simulink model "qdr_ct_test4"  (R2013b)
settings: Solver=FixedStepDiscrete  SolverMode=SingleTasking  StartTime=0.0  StopTime=1000.0  RelTol=1e-3
libraries: xbsIndex_r4 x636, casper_library_delays x8, xps_library x7, casper_library_misc x7
(part 1 of 8)
settings Model: Creator=franco  LastModifiedBy=root

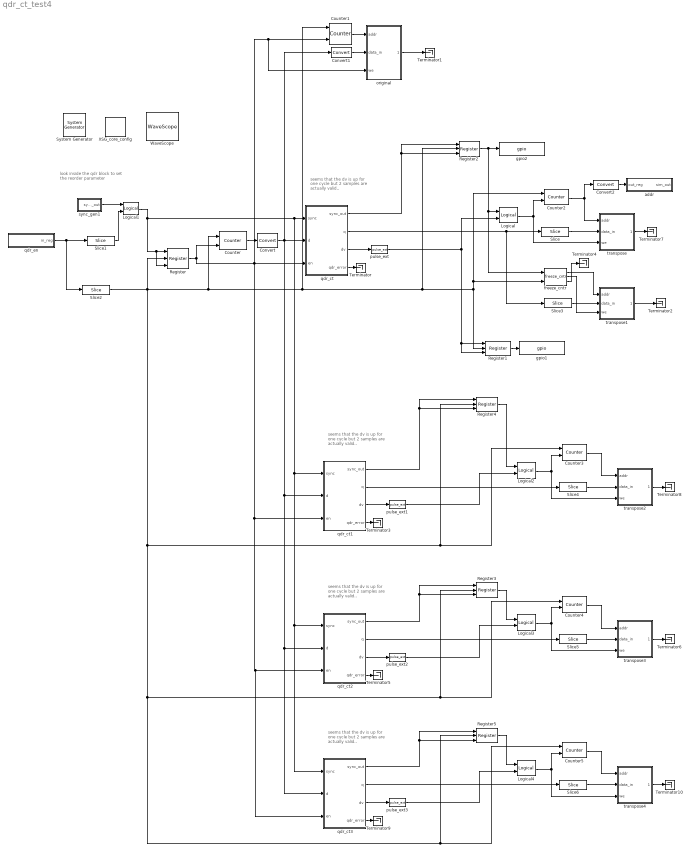
== system qdr_ct_test4 ==
  note: seems that the dv
      | is up for one cycle
      | but 2 samples are
      | actually valid..
  note: look inside the qdr block
      | to set the reorder parameter
  note: seems that the dv
      | is up for one cycle
      | but 2 samples are
      | actually valid..
  note: seems that the dv
      | is up for one cycle
      | but 2 samples are
      | actually valid..
  note: seems that the dv
      | is up for one cycle
      | but 2 samples are
      | actually valid..
  " System Generator" : xbsIndex_r4/ System Generator  Tag=genX  xilinxfamily=virtex6  part=xc6vsx475t  speed=-1  package=ff1759  synthesis_tool=XST  clock_wrapper=Clock Enables  directory=./qdr_ct_test/sysgen  proj_type=Project Navigator  Synth_file=XST Defaults  Impl_file=ISE Defaults  testbench=off  simulink_period=1  sysclk_period=7.4074  dcm_input_clock_period=100  incr_netlist=off  trim_vbits=Everywhere in SubSystem  dbl_ovrd=According to Block Masks  core_generation=According to Block Masks  run_coregen=off  deprecated_control=off  eval_field=0  block_type=sysgen
  Convert : xbsIndex_r4/Convert  gui_display_data_type=Fixed-point  arith_type=Unsigned  n_bits=72  bin_pt=0  float_type=Single  exp_bits=8  fraction_bits=24  quantization=Truncate  overflow=Wrap  en=off  latency=0  dbl_ovrd=off  pipeline=off  block_type=convert
  Convert1 : xbsIndex_r4/Convert  gui_display_data_type=Fixed-point  arith_type=Unsigned  n_bits=32  bin_pt=0  float_type=Single  exp_bits=8  fraction_bits=24  quantization=Truncate  overflow=Wrap  en=off  latency=0  dbl_ovrd=off  pipeline=off  block_type=convert
  Convert2 : xbsIndex_r4/Convert  gui_display_data_type=Fixed-point  arith_type=Unsigned  n_bits=32  bin_pt=0  float_type=Single  exp_bits=8  fraction_bits=24  quantization=Truncate  overflow=Wrap  en=off  latency=2  dbl_ovrd=off  pipeline=off  block_type=convert
      settings: block_version=11.4
  Counter{,1..5} (6 alike) : xbsIndex_r4/Counter  cnt_type=Free Running  cnt_to=Inf  operation=Up  start_count=0  cnt_by_val=1  arith_type=Unsigned  n_bits=16  bin_pt=0  load_pin=off  rst=on  en=on  explicit_period=on  period=1  dbl_ovrd=off  use_behavioral_HDL=off  implementation=Fabric  block_type=counter
  Logical{,1..4} (5 alike) : xbsIndex_r4/Logical  logical_function=AND  inputs=2  en=off  latency=0  precision=Full  arith_type=Unsigned  n_bits=16  bin_pt=0  align_bp=on  dbl_ovrd=off  block_type=logical
  Register{,1..5} (6 alike) : xbsIndex_r4/Register  init=0  rst=on  en=on  dbl_ovrd=off  block_type=register
  Slice{,3..6} (5 alike) : xbsIndex_r4/Slice  nbits=32  boolean_output=off  mode=Lower Bit Location + Width  bit1=0  base1=MSB of Input  bit0=0  base0=LSB of Input  dbl_ovrd=off  block_type=slice
  Slice1 : xbsIndex_r4/Slice  nbits=1  boolean_output=on  mode=Lower Bit Location + Width  bit1=0  base1=MSB of Input  bit0=0  base0=LSB of Input  dbl_ovrd=off  block_type=slice
  Slice2 : xbsIndex_r4/Slice  nbits=1  boolean_output=on  mode=Lower Bit Location + Width  bit1=0  base1=MSB of Input  bit0=1  base0=LSB of Input  dbl_ovrd=off  block_type=slice
  Terminator{,1..10} (11 alike) : Terminator
  WaveScope : xbsIndex_r4/WaveScope  block_type=wavescope
  XSG_core_config : xps_library/XSG_core_config  Tag=xps:xsg  hw_sys=ROACH2:sx475t  clk_src=sys_clk  ROACH_clk_src=sys_clk  ROACH2_clk_src=sys_clk  MKDIG_clk_src=sys_clk  clk_rate=135  sample_period=1  synthesis_tool=XST
  addr : Subsystem  Tag=xps:sw_reg  AncestorBlock=xps_library/software_register  mask(swreg){io_dir=To Processor, io_delay=0, sample_period=1, names=reg, bitwidths=32, bin_pts=0, arith_types=0, sim_port=on, show_format=on}
      mask prompts: io_dir "I/O direction"; io_delay "I/O delay"; sample_period "Sample period"; names "Bitfield names [msb...lsb]"; bitwidths "Bitfield widths"; bin_pts "Bitfield binary pts"; arith_types "Bitfield types, ufix=0, fix=1, bool=2"; sim_port "Provide sim input/output?"; show_format "Print format string?"
      mask help: A 32-bit software-accessible register. Can be divided into bitfields of varying widths and types using the fields in the block mask.
      mask init:
      | try
      |     swreg_init(gcb)
      | catch ex
      |     disp(sprintf('%s: %s', gcb, ex.message))
      |     errordlg(ex.message)
      | end
      settings: AttributesFormatString=1output:uf32.0 = 32 bits
      mask TypeOptions io_dir: To Processor | From Processor
      mask Callback io_dir:
      | mask_enables = get_param(gcb, 'MaskEnables');
      | mask_names = get_param(gcb, 'MaskNames');
      | if strcmp(get_param(gcb, 'io_dir'), 'To Processor'),
      |     mask_enables{ismember(mask_names, 'sample_period')} = 'off';
      | else
      |     mask_enables{ismember(mask_names, 'sample_period')} = 'on';
      | end
      | set_param(gcb, 'MaskEnables', mask_enables);
  freeze_cntr : casper_library_misc/freeze_cntr  CounterBits=16
  gpio1 : xps_library/gpio  Tag=xps:gpio  io_group=ROACH2:led  io_dir=out  arith_type=Boolean  bitwidth=1  bin_pt=0  bit_index=1  sample_period=1  use_single_ended=off  use_ddr=off  reg_iob=on  reg_clk_phase=0  termination=None
  gpio2 : xps_library/gpio  Tag=xps:gpio  io_group=ROACH2:led  io_dir=out  arith_type=Boolean  bitwidth=1  bin_pt=0  bit_index=0  sample_period=1  use_single_ended=off  use_ddr=off  reg_iob=on  reg_clk_phase=0  termination=None
  original : Subsystem  Tag=xps:bram  AncestorBlock=xps_library/Shared_BRAM  mask{arith_type=Unsigned, addr_width=16, data_width=32, reg_prim_output=off, reg_core_output=off, optimization=Minimum_Area, data_bin_pt=0, init_vals=[0:2^10-1], sample_rate=1}
      mask prompts: arith_type "Output Data Type"; addr_width "Address width"; data_width "Data Width"; reg_prim_output "Register Primitive Output"; reg_core_output "Register Core Output"; data_bin_pt "Data Binary Point"; init_vals "Initial values (simulation only)"; sample_rate "Sample rate"
      mask init:
      | shared_bram_mask;
      mask TypeOptions arith_type: Unsigned | Signed  (2's comp)
      mask TypeOptions data_width: 8 | 16 | 32 | 64 | 128
      mask TypeOptions optimization: Minimum_Area | Low_Power
  pulse_ext{,1..3} (4 alike) : casper_library_misc/pulse_ext  pulse_len=2
  qdr_ct : Subsystem  AncestorBlock=casper_library_reorder/qdr_ct  mask{idepth=8, odepth=8, which_qdr=qdr0, swap_input=no, output_order=in order, step_bits=0, custom_map=[1  15   5   7  10  14   6   0   8   9   2  13  12  11   4   3]}
      mask prompts: idepth "Input vector length (2^?)"; odepth "Output vector length (2^?)"; which_qdr "QDR SRAM chip"; swap_input "Swap input halves?"; output_order "Output column order"; step_bits "Interleave step (2^?)"; custom_map "Custom map"
      mask help:
      | Writes vectors in as rows in matrix and reads
      | out columns. Order in which columns read out
      | determined by 'Output column order' parameter.
      mask init:
      | if (strcmp(output_order, 'interleaved') == 1) && (step_bits > (idepth-1)) ,
      |     errmsg = sprintf('Can''t make step size (%i) bigger than (input vector bit size (%i) - 1)', step_bits, idepth);
      |     errordlg(errmsg);
      | end    
      | 
      | if strcmp(output_order, 'custom') && (...
      |         length(unique(custom_map)) ~= 2^idepth ||...
      |         ~isempty(find(custom_map < 0)) || ...
      |         ~isempty(find(custom_map > (2^idepth)-1))),
      |     disp('Custom map elements must be unique in range 0->2^(input vector)-1');
      |     return;
      | end
      | 
      | % set up output order (in order, interleaved, or custom)
      | map = 0 : (2^idepth)-1;
      | if strcmp(swap_input, 'yes'),
      |     map = [map((length(map)/2)+1:end), map(1:length(map)/2)];
      | end
      | if strcmp(output_order, 'interleaved'),
      |     index = zeros(1, 2^idepth);
      |     step_size = 2^(idepth-step_bits);
      |     for ctr = 0:(2^step_bits)-1,
      |         start = (ctr * step_size) + 1;
      |         finish = start + step_size - 1;
      |         index(start:finish) = ctr+1 : 2^step_bits : 2^idepth;
      |     end
      |     map = map(index);
      |     clear index;
      | elseif strcmp(output_order, 'custom'),
      |     map = map(custom_map+1);
      | end
      | 
      | %generate map so that two samples from same position in 
      | %subsequent input vectors are written into same address
      | map = reshape([map; 2^idepth+map], 1, 2^(idepth+1));
      | 
      | set_param([gcb, '/reorder'], ...
      |     'map', ['[',num2str(map),']']);
      | set_param([gcb, '/qdr'], 'which_qdr', which_qdr);
      mask TypeOptions which_qdr: qdr0 | qdr1 | qdr2 | qdr3
      mask TypeOptions swap_input: no | yes
      mask TypeOptions output_order: in order | interleaved | custom
  qdr_ct1 : Subsystem  AncestorBlock=casper_library_reorder/qdr_ct  mask{idepth=8, odepth=8, which_qdr=qdr1, swap_input=no, output_order=in order, step_bits=0, custom_map=[1  15   5   7  10  14   6   0   8   9   2  13  12  11   4   3]}
      mask prompts: idepth "Input vector length (2^?)"; odepth "Output vector length (2^?)"; which_qdr "QDR SRAM chip"; swap_input "Swap input halves?"; output_order "Output column order"; step_bits "Interleave step (2^?)"; custom_map "Custom map"
      mask help:
      | Writes vectors in as rows in matrix and reads
      | out columns. Order in which columns read out
      | determined by 'Output column order' parameter.
      mask init: same as qdr_ct_test4/qdr_ct
      mask TypeOptions which_qdr: qdr0 | qdr1 | qdr2 | qdr3
      mask TypeOptions swap_input: no | yes
      mask TypeOptions output_order: in order | interleaved | custom
  qdr_ct2 : Subsystem  AncestorBlock=casper_library_reorder/qdr_ct  mask{idepth=8, odepth=8, which_qdr=qdr2, swap_input=no, output_order=in order, step_bits=0, custom_map=[1  15   5   7  10  14   6   0   8   9   2  13  12  11   4   3]}
      mask prompts: idepth "Input vector length (2^?)"; odepth "Output vector length (2^?)"; which_qdr "QDR SRAM chip"; swap_input "Swap input halves?"; output_order "Output column order"; step_bits "Interleave step (2^?)"; custom_map "Custom map"
      mask help:
      | Writes vectors in as rows in matrix and reads
      | out columns. Order in which columns read out
      | determined by 'Output column order' parameter.
      mask init: same as qdr_ct_test4/qdr_ct
      mask TypeOptions which_qdr: qdr0 | qdr1 | qdr2 | qdr3
      mask TypeOptions swap_input: no | yes
      mask TypeOptions output_order: in order | interleaved | custom
  qdr_ct3 : Subsystem  AncestorBlock=casper_library_reorder/qdr_ct  mask{idepth=8, odepth=8, which_qdr=qdr3, swap_input=no, output_order=in order, step_bits=0, custom_map=[1  15   5   7  10  14   6   0   8   9   2  13  12  11   4   3]}
      mask prompts: idepth "Input vector length (2^?)"; odepth "Output vector length (2^?)"; which_qdr "QDR SRAM chip"; swap_input "Swap input halves?"; output_order "Output column order"; step_bits "Interleave step (2^?)"; custom_map "Custom map"
      mask help:
      | Writes vectors in as rows in matrix and reads
      | out columns. Order in which columns read out
      | determined by 'Output column order' parameter.
      mask init: same as qdr_ct_test4/qdr_ct
      mask TypeOptions which_qdr: qdr0 | qdr1 | qdr2 | qdr3
      mask TypeOptions swap_input: no | yes
      mask TypeOptions output_order: in order | interleaved | custom
  qdr_en : Subsystem  Tag=xps:sw_reg  AncestorBlock=xps_library/software_register  mask(swreg){io_dir=From Processor, io_delay=0, sample_period=1, names=reg, bitwidths=32, bin_pts=0, arith_types=0, sim_port=off, show_format=off}
      mask prompts: io_dir "I/O direction"; io_delay "I/O delay"; sample_period "Sample period"; names "Bitfield names [msb...lsb]"; bitwidths "Bitfield widths"; bin_pts "Bitfield binary pts"; arith_types "Bitfield types, ufix=0, fix=1, bool=2"; sim_port "Provide sim input/output?"; show_format "Print format string?"
      mask help: A 32-bit software-accessible register. Can be divided into bitfields of varying widths and types using the fields in the block mask.
      mask init:
      | try
      |     swreg_init(gcb)
      | catch ex
      |     disp(sprintf('%s: %s', gcb, ex.message))
      |     errordlg(ex.message)
      | end
      settings: AttributesFormatString=1input
      mask TypeOptions io_dir: To Processor | From Processor
      mask Callback io_dir:
      | mask_enables = get_param(gcb, 'MaskEnables');
      | mask_names = get_param(gcb, 'MaskNames');
      | if strcmp(get_param(gcb, 'io_dir'), 'To Processor'),
      |     mask_enables{ismember(mask_names, 'sample_period')} = 'off';
      | else
      |     mask_enables{ismember(mask_names, 'sample_period')} = 'on';
      | end
      | set_param(gcb, 'MaskEnables', mask_enables);
  sync_gen1 : Subsystem  AncestorBlock=casper_library_misc/sync_gen  mask(sync_gen){sim_acc_len=1, fft_size=2^16, fft_simult_inputs=1, pfb_fir_taps=1, reorder_vec=9, scale=1}
      mask prompts: sim_acc_len "Simulation Accumulation Length"; fft_size "FFT Size"; fft_simult_inputs "Simultaneous Inputs (FFT)"; pfb_fir_taps "Taps in pfb_fir (use 1 if no pfb_fir)"; reorder_vec "Reorder Orders (e.g. [2 2 2])"
      mask help:
      | This block computes the sync period based on system parameters as
      | described in Casper memo.  Detailed descritions of the block's
      | variables can be found in the 'Block Documentation' section of
      | the CASPER wiki.
      mask init:
      | sync_gen_init(gcb, ...
      |     'sim_acc_len', sim_acc_len, ...
      |     'fft_size', fft_size, ...
      |     'fft_simult_inputs', fft_simult_inputs,...
      |     'pfb_fir_taps', pfb_fir_taps, ...
      |     'reorder_vec', reorder_vec, ...
      |     'scale', scale);
      settings: AttributesFormatString=sim_sync_period=589824
      mask Help:
      | SyncPeriod=LCM(reorder_vec)*(acc_num)*(pfb_fir_len)*(fft_size/fft_simult_inputs)
      | 
      | See CASPER sync pulse memo for more details.
  transpose : Subsystem  Tag=xps:bram  AncestorBlock=xps_library/Shared_BRAM  mask{arith_type=Unsigned, addr_width=16, data_width=32, reg_prim_output=off, reg_core_output=off, optimization=Minimum_Area, data_bin_pt=0, init_vals=[0:2^10-1], sample_rate=1}
      mask prompts: arith_type "Output Data Type"; addr_width "Address width"; data_width "Data Width"; reg_prim_output "Register Primitive Output"; reg_core_output "Register Core Output"; data_bin_pt "Data Binary Point"; init_vals "Initial values (simulation only)"; sample_rate "Sample rate"
      mask init:
      | shared_bram_mask;
      mask TypeOptions arith_type: Unsigned | Signed  (2's comp)
      mask TypeOptions data_width: 8 | 16 | 32 | 64 | 128
      mask TypeOptions optimization: Minimum_Area | Low_Power
  transpose1 : Subsystem  Tag=xps:bram  AncestorBlock=xps_library/Shared_BRAM  mask{arith_type=Unsigned, addr_width=16, data_width=32, reg_prim_output=off, reg_core_output=off, optimization=Minimum_Area, data_bin_pt=0, init_vals=[0:2^10-1], sample_rate=1}
      mask prompts: arith_type "Output Data Type"; addr_width "Address width"; data_width "Data Width"; reg_prim_output "Register Primitive Output"; reg_core_output "Register Core Output"; data_bin_pt "Data Binary Point"; init_vals "Initial values (simulation only)"; sample_rate "Sample rate"
      mask init:
      | shared_bram_mask;
      mask TypeOptions arith_type: Unsigned | Signed  (2's comp)
      mask TypeOptions data_width: 8 | 16 | 32 | 64 | 128
      mask TypeOptions optimization: Minimum_Area | Low_Power
  transpose2 : Subsystem  Tag=xps:bram  AncestorBlock=xps_library/Shared_BRAM  mask{arith_type=Unsigned, addr_width=16, data_width=32, reg_prim_output=off, reg_core_output=off, optimization=Minimum_Area, data_bin_pt=0, init_vals=[0:2^10-1], sample_rate=1}
      mask prompts: arith_type "Output Data Type"; addr_width "Address width"; data_width "Data Width"; reg_prim_output "Register Primitive Output"; reg_core_output "Register Core Output"; data_bin_pt "Data Binary Point"; init_vals "Initial values (simulation only)"; sample_rate "Sample rate"
      mask init:
      | shared_bram_mask;
      mask TypeOptions arith_type: Unsigned | Signed  (2's comp)
      mask TypeOptions data_width: 8 | 16 | 32 | 64 | 128
      mask TypeOptions optimization: Minimum_Area | Low_Power
  transpose3 : Subsystem  Tag=xps:bram  AncestorBlock=xps_library/Shared_BRAM  mask{arith_type=Unsigned, addr_width=16, data_width=32, reg_prim_output=off, reg_core_output=off, optimization=Minimum_Area, data_bin_pt=0, init_vals=[0:2^10-1], sample_rate=1}
      mask prompts: arith_type "Output Data Type"; addr_width "Address width"; data_width "Data Width"; reg_prim_output "Register Primitive Output"; reg_core_output "Register Core Output"; data_bin_pt "Data Binary Point"; init_vals "Initial values (simulation only)"; sample_rate "Sample rate"
      mask init:
      | shared_bram_mask;
      mask TypeOptions arith_type: Unsigned | Signed  (2's comp)
      mask TypeOptions data_width: 8 | 16 | 32 | 64 | 128
      mask TypeOptions optimization: Minimum_Area | Low_Power
  transpose4 : Subsystem  Tag=xps:bram  AncestorBlock=xps_library/Shared_BRAM  mask{arith_type=Unsigned, addr_width=16, data_width=32, reg_prim_output=off, reg_core_output=off, optimization=Minimum_Area, data_bin_pt=0, init_vals=[0:2^10-1], sample_rate=1}
      mask prompts: arith_type "Output Data Type"; addr_width "Address width"; data_width "Data Width"; reg_prim_output "Register Primitive Output"; reg_core_output "Register Core Output"; data_bin_pt "Data Binary Point"; init_vals "Initial values (simulation only)"; sample_rate "Sample rate"
      mask init:
      | shared_bram_mask;
      mask TypeOptions arith_type: Unsigned | Signed  (2's comp)
      mask TypeOptions data_width: 8 | 16 | 32 | 64 | 128
      mask TypeOptions optimization: Minimum_Area | Low_Power
  wires:
  Counter/1 -> Convert/1
  Convert/1 -> qdr_ct3/2(d), qdr_ct2/2(d), qdr_ct1/2(d), qdr_ct/2(d), Convert1/1
  qdr_ct/2(q) -> Slice3/1, Slice/1
  Counter2/1 -> transpose/1(addr), Convert2/1
  transpose/1(data_out) -> Terminator7/1
  Slice/1 -> transpose/2(data_in)
  qdr_en/1(in_reg) -> Slice2/1, Slice1/1
  Counter1/1 -> original/1(addr)
  original/1(data_out) -> Terminator1/1
  Convert1/1 -> original/2(data_in)
  Register1/1 -> gpio1/1
  qdr_ct/4(qdr_error) -> Terminator/1
  Register2/1 -> gpio2/1, Logical/1, freeze_cntr/1
  qdr_ct/1(sync_out) -> Register2/3, Register2/1
  Convert2/1 -> addr/1(out_reg)
  transpose1/1(data_out) -> Terminator2/1
  Slice3/1 -> transpose1/2(data_in)
  freeze_cntr/1 -> transpose1/1(addr)
  freeze_cntr/2 -> transpose1/3(we)
  freeze_cntr/3 -> Terminator4/1
  qdr_ct/3(dv) -> pulse_ext/1
  Logical/1 -> transpose/3(we), Counter2/2
  Slice1/1 -> Logical1/2
  Register/1 -> qdr_ct3/3(en), qdr_ct2/3(en), qdr_ct1/3(en), original/3(we), Counter1/2, qdr_ct/3(en), Counter/2
  sync_gen1/1(sync_out) -> Logical1/1
  Logical1/1 -> qdr_ct3/1(sync), qdr_ct2/1(sync), qdr_ct1/1(sync), qdr_ct/1(sync), Register/3, Register/1
  pulse_ext/1 -> Logical/2, Register1/3, Register1/1
  qdr_ct1/2(q) -> Slice4/1
  Counter3/1 -> transpose2/1(addr)
  transpose2/1(data_out) -> Terminator8/1
  Slice4/1 -> transpose2/2(data_in)
  qdr_ct1/4(qdr_error) -> Terminator3/1
  Register4/1 -> Logical2/1
  qdr_ct1/1(sync_out) -> Register4/3, Register4/1
  qdr_ct1/3(dv) -> pulse_ext1/1
  Logical2/1 -> transpose2/3(we), Counter3/2
  pulse_ext1/1 -> Logical2/2
  qdr_ct2/2(q) -> Slice5/1
  Counter4/1 -> transpose3/1(addr)
  transpose3/1(data_out) -> Terminator6/1
  Slice5/1 -> transpose3/2(data_in)
  qdr_ct2/4(qdr_error) -> Terminator5/1
  Register3/1 -> Logical3/1
  qdr_ct2/1(sync_out) -> Register3/3, Register3/1
  qdr_ct2/3(dv) -> pulse_ext2/1
  Logical3/1 -> transpose3/3(we), Counter4/2
  pulse_ext2/1 -> Logical3/2
  qdr_ct3/2(q) -> Slice6/1
  Counter5/1 -> transpose4/1(addr)
  transpose4/1(data_out) -> Terminator10/1
  Slice6/1 -> transpose4/2(data_in)
  qdr_ct3/4(qdr_error) -> Terminator9/1
  Slice2/1 -> Counter5/1, Register5/2, Register3/2, Counter4/1, Counter3/1, Register4/2, Register/2, freeze_cntr/2, Counter2/1, Register1/2, Register2/2, Counter1/1, Counter/1
  Register5/1 -> Logical4/1
  qdr_ct3/1(sync_out) -> Register5/3, Register5/1
  qdr_ct3/3(dv) -> pulse_ext3/1
  Logical4/1 -> transpose4/3(we), Counter5/2
  pulse_ext3/1 -> Logical4/2

== system qdr_ct_test4/addr ==
  out_reg : Inport
  assert_reg : xbsIndex_r4/Assert  assert_type=on  type_source=Explicitly  gui_display_data_type=Fixed-point  arith_type=Unsigned  n_bits=32  bin_pt=0  preci_type=Single  exp_width=8  frac_width=24  assert_rate=off  rate_source=Explicitly  period=1  output_port=on  block_type=assert
  cast_gw : xbsIndex_r4/Convert  gui_display_data_type=Fixed-point  arith_type=Unsigned  n_bits=32  bin_pt=0  float_type=Single  exp_bits=8  fraction_bits=24  quantization=Truncate  overflow=Wrap  en=off  latency=0  dbl_ovrd=off  pipeline=off  block_type=convert
  io_delay : xbsIndex_r4/Delay  rst=off  infoeditControl=Selection of Reset will increase slice count due to use of real FFs and instead of SRLs  en=off  latency=0  dbl_ovrd=off  reg_retiming=on  block_type=delay
  qdr_ct_test_addr_user_data_in : xbsIndex_r4/Gateway Out  inherit_from_input=off  hdl_port=on  timing_constraint=None  locs_specified=off  LOCs={}  UseAsDAC=off  DACChannel='1'  block_type=gatewayout
  reint1 : xbsIndex_r4/Reinterpret  force_arith_type=on  arith_type=Unsigned  force_bin_pt=on  bin_pt=0  block_type=reinterpret
  sim_out : Outport
  wires:
  io_delay/1 -> cast_gw/1
  cast_gw/1 -> qdr_ct_test_addr_user_data_in/1
  qdr_ct_test_addr_user_data_in/1 -> sim_out/1
  out_reg/1 -> assert_reg/1
  assert_reg/1 -> reint1/1
  reint1/1 -> io_delay/1

== system qdr_ct_test4/original ==
  addr : Inport
  data_in : Inport  Port=2
  we : Inport  Port=3
  calc_add : Subsystem  mask{data_width=32, addr_width=16, sample_rate=sample_rate}
      mask prompts: data_width "data width"; addr_width "address width"; sample_rate "sample rate"
  convert_addr : xbsIndex_r4/Convert  gui_display_data_type=Fixed-point  arith_type=Unsigned  n_bits=addr_width  bin_pt=0  float_type=Single  exp_bits=8  fraction_bits=24  quantization=Truncate  overflow=Wrap  en=off  latency=0  dbl_ovrd=off  pipeline=off  block_type=convert
      settings: xl_area=[0, 0, 0, 0, 0, 0, 0]
  convert_din1 : xbsIndex_r4/Convert  gui_display_data_type=Fixed-point  arith_type=Unsigned  n_bits=32  bin_pt=0  float_type=Single  exp_bits=8  fraction_bits=24  quantization=Truncate  overflow=Wrap  en=off  latency=0  dbl_ovrd=off  pipeline=off  block_type=convert
      settings: xl_area=[0, 0, 0, 0, 0, 0, 0]
  convert_we : xbsIndex_r4/Convert  gui_display_data_type=Fixed-point  arith_type=Unsigned  n_bits=1  bin_pt=0  float_type=Single  exp_bits=8  fraction_bits=24  quantization=Truncate  overflow=Wrap  en=off  latency=0  dbl_ovrd=off  pipeline=off  block_type=convert
      settings: xl_area=[0, 0, 0, 0, 0, 0, 0]
  mem : Subsystem
  munge_in : Subsystem  AncestorBlock=casper_library_flow_control/munge  mask(munge){divisions=1, div_size=32, order=[0], arith_type_out=Unsigned, bin_pt_out=0}
      mask prompts: divisions "Number of divisions"; div_size "Division size (bits)"; order "Division packing order"; arith_type_out "Output arithmetic type"; bin_pt_out "Output binary point"
      mask help: Splits an input bus into the specified number of divisions and then recombines them in the order specified (most significant division = 0,least = number divisions-1)
      mask init:
      | munge_init(gcb, ...
      |     'divisions', divisions, ...
      |     'div_size', div_size, ...
      |     'order', order, ...
      |     'arith_type_out', arith_type_out, ...
      |     'bin_pt_out', bin_pt_out);
      settings: AttributesFormatString=|
      | split:32
      | join:0
      | Unsigned [32,0]
      mask TypeOptions arith_type_out: Unsigned | Signed  (2's comp) | Floating-point
  munge_out : Subsystem  AncestorBlock=casper_library_flow_control/munge  mask(munge){divisions=1, div_size=32, order=[0], arith_type_out=Unsigned, bin_pt_out=0}
      mask prompts: divisions "Number of divisions"; div_size "Division size (bits)"; order "Division packing order"; arith_type_out "Output arithmetic type"; bin_pt_out "Output binary point"
      mask help: Splits an input bus into the specified number of divisions and then recombines them in the order specified (most significant division = 0,least = number divisions-1)
      mask init:
      | munge_init(gcb, ...
      |     'divisions', divisions, ...
      |     'div_size', div_size, ...
      |     'order', order, ...
      |     'arith_type_out', arith_type_out, ...
      |     'bin_pt_out', bin_pt_out);
      settings: AttributesFormatString=|
      | split:32
      | join:0
      | Unsigned [32,0]
      mask TypeOptions arith_type_out: Unsigned | Signed  (2's comp) | Floating-point
  qdr_ct_test_original_addr : xbsIndex_r4/Gateway Out  inherit_from_input=off  hdl_port=on  timing_constraint=None  locs_specified=off  LOCs={'A5','B9','A9','C1','A3','G6','E9','A6','A7','A8','B8','B1','B3','D9','B5','B4','B6','C2'}  UseAsDAC=off  DACChannel='1'  block_type=gatewayout
      settings: infoedit="Gateway out block.  Converts Xilinx fixed point inputs into ouputs of type Simulink integer, double, or fixed point.<P><P>Hardware notes:  In hardware these blocks become top level output ports or are discarded, depending on how they are configured."  xl_area=[0, 0, 0, 0, 0, 0, 0]  sginterface={'Nallatech'=>{'xdspkit'=>{'non_memory_mapped_port'=>'uprev_Shared_BRAM_addr'}},'Xilinx'=>{'jtaghwcosim'=>{'non_memory_mapped_port'=>'uprev_Shared_BRAM_addr'},'xdspkit'=>{'non_memory_mapped_port'=>'uprev_Shared_BRAM_addr'}}}
  qdr_ct_test_original_data_in : xbsIndex_r4/Gateway Out  inherit_from_input=off  hdl_port=on  timing_constraint=None  locs_specified=off  LOCs={'B21','B22','A22','B23','B19','C19','A20','A21','A23','B24','A24','A25','E18','D18','C18','B18'}  UseAsDAC=off  DACChannel='1'  block_type=gatewayout
      settings: infoedit="Gateway out block.  Converts Xilinx fixed point inputs into ouputs of type Simulink integer, double, or fixed point.<P><P>Hardware notes:  In hardware these blocks become top level output ports or are discarded, depending on how they are configured."  xl_area=[0, 0, 0, 0, 0, 0, 0]  sginterface={'Nallatech'=>{'xdspkit'=>{'non_memory_mapped_port'=>'uprev_Shared_BRAM_data_in'}},'Xilinx'=>{'jtaghwcosim'=>{'non_memory_mapped_port'=>'uprev_Shared_BRAM_data_in'},'xdspkit'=>{'non_memory_mapped_port'=>'uprev_Shared_BRAM_data_in'}}}
  qdr_ct_test_original_data_out : xbsIndex_r4/Gateway In  gui_display_data_type=Fixed-point  arith_type=Unsigned  n_bits=32  bin_pt=0  preci_type=Single  exp_width=8  frac_width=24  quantization=Truncate  overflow=Wrap  period=sample_rate  dbl_ovrd=off  timing_constraint=None  locs_specified=off  LOCs={}  UseAsADC=off  ADCChannel='1'  inherit_from_input=off  hdl_port=on  block_type=gatewayin
      settings: xl_area=[0, 0, 0, 0, 0, 0, 0]
  qdr_ct_test_original_we : xbsIndex_r4/Gateway Out  inherit_from_input=off  hdl_port=on  timing_constraint=None  locs_specified=off  LOCs={'A14'}  UseAsDAC=off  DACChannel='1'  block_type=gatewayout
      settings: infoedit="Gateway out block.  Converts Xilinx fixed point inputs into ouputs of type Simulink integer, double, or fixed point.<P><P>Hardware notes:  In hardware these blocks become top level output ports or are discarded, depending on how they are configured."  xl_area=[0, 0, 0, 0, 0, 0, 0]
  data_out : Outport
  wires:
  convert_addr/1 -> qdr_ct_test_original_addr/1
  convert_din1/1 -> qdr_ct_test_original_data_in/1
  data_in/1 -> munge_in/1(din)
  calc_add/1(out) -> convert_addr/1
  qdr_ct_test_original_we/1 -> mem/3(In3)
  qdr_ct_test_original_data_in/1 -> mem/2(In2)
  qdr_ct_test_original_addr/1 -> mem/1(In1)
  convert_we/1 -> qdr_ct_test_original_we/1
  qdr_ct_test_original_data_out/1 -> munge_out/1(din)
  mem/1(Out1) -> qdr_ct_test_original_data_out/1
  addr/1 -> calc_add/1(in)
  we/1 -> convert_we/1
  munge_out/1(dout) -> data_out/1
  munge_in/1(dout) -> convert_din1/1

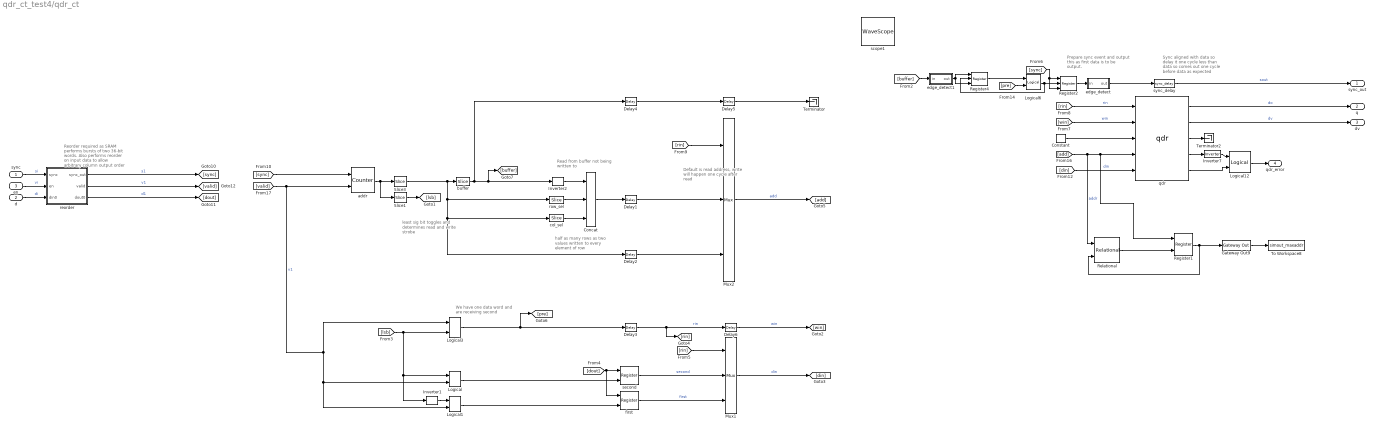
== system qdr_ct_test4/qdr_ct ==
  note: half as many rows
      | as two values
      | written to every
      | element of row
  note: Read from buffer
      | not being
      | written to
  note: Default is read address,
      | write will happen one
      | cycle after read
  note: We have one data word
      | and are receiving second
  note: least sig bit toggles
      | and determines read
      | and write strobe
  note: Sync aligned with data so
      | delay it one cycle less
      | than data so comes out one
      | cycle before data as
      | expected
  note: Prepare sync event and output
      | this as first data is to be output.
  note: Reorder required as SRAM performs
      | bursts of two 36-bit words.
      | Also performs reorder on input
      | data to allow arbitrary column
      | output order
  sync : Inport
  d : Inport  Port=2
  en : Inport  Port=3
  Concat : xbsIndex_r4/Concat  num_inputs=3  dbl_ovrd=off  block_type=concat
      settings: block_version=10.1.3
  Constant : xbsIndex_r4/Constant  const=255  gui_display_data_type=Fixed-point  arith_type=Unsigned  n_bits=8  bin_pt=0  preci_type=Single  exp_width=8  frac_width=24  explicit_period=on  period=1  equ=P=C  opselect=C  inp2=PCIN>>17  opr=+  inp1=P  carry=CIN  dbl_ovrd=off  block_type=constant
  Delay{1..6} (6 alike) : xbsIndex_r4/Delay  rst=off  infoeditControl=Selection of Reset will increase slice count due to use of real FFs and instead of SRLs  en=off  latency=1  dbl_ovrd=off  reg_retiming=on  block_type=delay
      settings: block_version=11.4
  Gateway Out9 : xbsIndex_r4/Gateway Out  inherit_from_input=off  hdl_port=off  timing_constraint=None  locs_specified=off  LOCs={}  UseAsDAC=off  DACChannel='1'  block_type=gatewayout
      settings: infoedit="Gateway out block.  Converts Xilinx fixed point inputs into ouputs of type Simulink integer, double, or fixed point.<br><br>Hardware notes:  In hardware these blocks become top level output ports or are discarded, depending on how they are configured."  block_version=11.4
  Inverter1 : xbsIndex_r4/Inverter  en=off  latency=0  dbl_ovrd=off  block_type=inv
  Inverter2 : xbsIndex_r4/Inverter  en=off  latency=0  dbl_ovrd=off  block_type=inv
  Inverter7 : xbsIndex_r4/Inverter  en=off  latency=0  dbl_ovrd=off  block_type=inv
      settings: block_version=11.4
  Logical{,1,3,6} (4 alike) : xbsIndex_r4/Logical  logical_function=AND  inputs=2  en=off  latency=0  precision=Full  arith_type=Unsigned  n_bits=16  bin_pt=0  align_bp=on  dbl_ovrd=off  block_type=logical
      settings: block_version=11.4
  Logical12 : xbsIndex_r4/Logical  logical_function=OR  inputs=2  en=off  latency=1  precision=Full  arith_type=Unsigned  n_bits=8  bin_pt=2  align_bp=on  dbl_ovrd=off  block_type=logical
      settings: xl_area=[0, 0, 0, 0, 0, 0, 0]
  Mux1 : xbsIndex_r4/Mux  inputs=2  en=off  latency=1  precision=Full  arith_type=Unsigned  n_bits=16  bin_pt=14  quantization=Truncate  overflow=Wrap  dbl_ovrd=off  block_type=mux
      settings: block_version=11.4
  Mux2 : xbsIndex_r4/Mux  inputs=2  en=off  latency=1  precision=Full  arith_type=Unsigned  n_bits=16  bin_pt=14  quantization=Truncate  overflow=Wrap  dbl_ovrd=off  block_type=mux
      settings: block_version=11.4
  Register1 : xbsIndex_r4/Register  init=0  rst=off  en=on  dbl_ovrd=off  block_type=register
      settings: block_version=11.4
  Register2 : xbsIndex_r4/Register  init=0  rst=on  en=on  dbl_ovrd=off  block_type=register
      settings: block_version=11.4
  Register4 : xbsIndex_r4/Register  init=0  rst=on  en=on  dbl_ovrd=off  block_type=register
      settings: block_version=11.4
  Relational : xbsIndex_r4/Relational  mode=a>b  en=off  latency=0  dbl_ovrd=off  block_type=relational
  Slice1 : xbsIndex_r4/Slice  nbits=1  boolean_output=on  mode=Lower Bit Location + Width  bit1=0  base1=MSB of Input  bit0=0  base0=LSB of Input  dbl_ovrd=off  block_type=slice
      settings: block_version=10.1.3
  Slice3 : xbsIndex_r4/Slice  nbits=(idepth + odepth + 1) - 1  boolean_output=off  mode=Upper Bit Location + Width  bit1=0  base1=MSB of Input  bit0=0  base0=LSB of Input  dbl_ovrd=off  block_type=slice
      settings: block_version=10.1.3
  Terminator : Terminator
  Terminator2 : Terminator
  To Workspace8 : ToWorkspace  VariableName=simout_maxaddr  SampleTime=-1  SaveFormat=Structure
      settings: MaxDataPoints=1
  addr : xbsIndex_r4/Counter  cnt_type=Free Running  cnt_to=Inf  operation=Up  start_count=0  cnt_by_val=1  arith_type=Unsigned  n_bits=(idepth + odepth + 1)  bin_pt=0  load_pin=off  rst=on  en=on  explicit_period=on  period=1  dbl_ovrd=off  use_behavioral_HDL=on  implementation=Fabric  use_rpm=off  block_type=counter
  buffer : xbsIndex_r4/Slice  nbits=1  boolean_output=on  mode=Upper Bit Location + Width  bit1=0  base1=MSB of Input  bit0=0  base0=LSB of Input  dbl_ovrd=off  block_type=slice
      settings: block_version=10.1.3
  col_sel : xbsIndex_r4/Slice  nbits=idepth  boolean_output=off  mode=Lower Bit Location + Width  bit1=0  base1=MSB of Input  bit0=odepth-1  base0=LSB of Input  dbl_ovrd=off  block_type=slice
      settings: block_version=10.1.3
  edge_detect : Subsystem  AncestorBlock=casper_library_misc/edge_detect  mask(edge_detect){edge=Falling, polarity=Active High, x_in=[0 0.08 0.08 0.16 0.16 0.24 0.24 0.32 0.32 0.4], y_in=[1  1 -1 -1 -1 -1 -1 -1 -1 -1], x_out=[0.6 0.68 0.68 0.76 0.76 0.84 0.84 0.92 0.92 1], y_out=[-1 -1  1  1 -1 -1 -1 -1 -1 -1]}
      mask prompts: edge "Edge Type"; polarity "Output Polarity"; x_in "Input X Positions"; y_in "Input Y Positions"; x_out "Output X Positions"; y_out "Output Y Positions"
      mask help: Output is active for one-cycle after each edge of the specified type (i.e. rising, falling or both).
      mask init:
      | edge_detect_init(gcb,...
      |     'edge',edge,...
      |     'polarity',polarity,...
      |     'x_in',x_in,...
      |     'x_out',x_out,...
      |     'y_in',y_in,...
      |     'y_out',y_out);
      | 
      | x_in_num=str2num(getfield(getfield(get_param(gcb,'UserData'),'parameters'),'x_in'));
      | x_out_num=str2num(getfield(getfield(get_param(gcb,'UserData'),'parameters'),'x_out'));
      | y_in_num=str2num(getfield(getfield(get_param(gcb,'UserData'),'parameters'),'y_in'));
      | y_out_num=str2num(getfield(getfield(get_param(gcb,'UserData'),'parameters'),'y_out'));
      settings: AttributesFormatString=|
      | falling edges
      | active high
      mask Help: Output is active for one-cycle after each edge of the specified type (i.e. rising, falling, or both).  Latency is zero.
      mask TypeOptions edge: Rising | Falling | Both
      mask TypeOptions polarity: Active High | Active Low
      mask Display:
      | plot(x_in_num,0.5+y_in_num*0.2);
      | plot(x_out_num,0.5+y_out_num*0.2);
  edge_detect1 : Subsystem  AncestorBlock=casper_library_misc/edge_detect  mask(edge_detect){edge=Rising, polarity=Active High, x_in=[0 0.08 0.08 0.16 0.16 0.24 0.24 0.32 0.32 0.4], y_in=[-1 -1  1  1  1  1  1  1  1  1], x_out=[0.6 0.68 0.68 0.76 0.76 0.84 0.84 0.92 0.92 1], y_out=[-1 -1  1  1 -1 -1 -1 -1 -1 -1]}
      mask prompts: edge "Edge Type"; polarity "Output Polarity"; x_in "Input X Positions"; y_in "Input Y Positions"; x_out "Output X Positions"; y_out "Output Y Positions"
      mask help: Output is active for one-cycle after each edge of the specified type (i.e. rising, falling or both).
      mask init: same as qdr_ct_test4/qdr_ct/edge_detect
      settings: AttributesFormatString=|
      | rising edges
      | active high
      mask Help: Output is active for one-cycle after each edge of the specified type (i.e. rising, falling, or both).  Latency is zero.
      mask TypeOptions edge: Rising | Falling | Both
      mask TypeOptions polarity: Active High | Active Low
      mask Display:
      | plot(x_in_num,0.5+y_in_num*0.2);
      | plot(x_out_num,0.5+y_out_num*0.2);
  first : xbsIndex_r4/Register  init=0  rst=off  en=on  dbl_ovrd=off  block_type=register
      settings: block_version=11.4
  qdr : xps_library/qdr  Tag=xps:qdr  which_qdr=qdr0  qdr_awidth=20  use_sniffer=on
      link override convert_data_in1: n_bits=72
      link override insert_parity: bitexpr=b = {a[71:0]}  arith_type1=Unsigned  arith_type2=Unsigned  arith_type3=Unsigned  arith_type4=Unsigned
  reorder : Subsystem  AncestorBlock=casper_library_reorder/reorder  mask(reorder){map=[0  256    1  257    2  258    3  259    4  260    5  261    6  262    7  263    8  264    9  265   10  266   11  267   12  268   13  269   14  270   15  271   16  272   17  273   18  274   19  275   20  276   21  277   22  278   23  279   24  280   25  281   26  282   27  283   28  284   29  285   30  286   31  287   32  288   33  289   34  290   35  291   36  292   37  293   38  294   39  295   40  296   41  297   42  298   43  299   44  300   45  301   46  302   47  303   48  304   49  305   50  306   51  307   52  308   53  309   54  310   55  311   56  312   57  313   58  314   59  315   60  316   61  317   62  318   63  319   64  320   65  321   66  322   67  323   68  324   69  325   70  326   71  327   72  328   73  329   74  330   75  331   76  332   77  333   78  334   79  335   80  336   81  337   82  338   83  339   84  340   85  341   86  342   87  343   88  344   89  345   90  346   91  347   92  348   93  349   94  350   95  351   96  352   97  353   98  354   99  355  100  356  101  357  102  358  103  359  104  360  105  361  106  362  107  363  108  364  109  365  110  366  111  367  112  368  113  369  114  370  115  371  116  372  117  373  118  374  119  375  120  376  121  377  122  378  123  379  124  380  125  381  126  382  127  383  128  384  129  385  130  386  131  387  132  388  133  389  134  390  135  391  136  392  137  393  138  394  139  395  140  396  141  397  142  398  143  399  144  400  145  401  146  402  147  403  148  404  149  405  150  406  151  407  152  408  153  409  154  410  155  411  156  412  157  413  158  414  159  415  160  416  161  417  162  418  163  419  164  420  165  421  166  422  167  423  168  424  169  425  170  426  171  427  172  428  173  429  174  430  175  431  176  432  177  433  178  434  179  435  180  436  181  437  182  438  183  439  184  440  185  441  186  442  187  443  188  444  189  445  190  446  191  447  192  448  193  449  194  450  195  451  196  452  197  453  198  454  199  455  200  456  201  457  202  458  203  459  204  460  205  461  206  462  207  463  208  464  209  465  210  466  211  467  212  468  213  469  214  470  215  471  216  472  217  473  218  474  219  475  220  476  221  477  222  478  223  479  224  480  225  481  226  482  227  483  228  484  229  485  230  486  231  487  232  488  233  489  234  490  235  491  236  492  237  493  238  494  239  495  240  496  241  497  242  498  243  499  244  500  245  501  246  502  247  503  248  504  249  505  250  506  251  507  252  508  253  509  254  510  255  511], n_bits=0, n_inputs=1, bram_latency=3, map_latency=2, fanout_latency=0, double_buffer=0, bram_map=on}
      mask prompts: map "Output Order:"; n_bits "Data width in"; n_inputs "Number of inputs"; bram_latency "BRAM Latency"; map_latency "Map Latency"; fanout_latency "Fanout latency"; double_buffer "Double Buffer"; bram_map "Use BlockRAM for Map"
      mask init:
      | reorder_init(gcb, ...
      |     'map', map, ...
      |     'n_bits', n_bits, ...
      |     'n_inputs', n_inputs, ...
      |     'bram_latency', bram_latency, ...
      |     'map_latency', map_latency, ...
      |     'fanout_latency', fanout_latency, ...
      |     'double_buffer', double_buffer, ...
      |     'bram_map', bram_map);
      settings: AttributesFormatString=order=9
      mask Help: eval('xlWeb(''http://casper.berkeley.edu/wiki/Reorder'')')
  row_sel : xbsIndex_r4/Slice  nbits=odepth-1  boolean_output=off  mode=Lower Bit Location + Width  bit1=0  base1=MSB of Input  bit0=0  base0=LSB of Input  dbl_ovrd=off  block_type=slice
      settings: block_version=10.1.3
  scope1 : xbsIndex_r4/WaveScope  block_type=wavescope
      settings: block_version=11.4
  second : xbsIndex_r4/Register  init=0  rst=off  en=on  dbl_ovrd=off  block_type=register
      settings: block_version=11.4
  sync_delay : casper_library_delays/sync_delay  DelayLen=10-1
  sync_out : Outport
  q : Outport  Port=2
  dv : Outport  Port=3
  qdr_error : Outport  Port=4
  wires:
  reorder/3(dout0) -> [dout]  "d1"
  reorder/2(valid) -> [valid]  "v1"
  reorder/1(sync_out) -> [sync]  "s1"
  [sync] -> addr/1
  Register1/1 -> Relational/2, Gateway Out9/1
  Relational/1 -> Register1/2
  Gateway Out9/1 -> To Workspace8/1
  qdr/2 -> dv/1  "dv"
  qdr/1 -> q/1  "do"
  sync_delay/1 -> sync_out/1  "sout"
  Logical12/1 -> qdr_error/1
  Inverter7/1 -> Logical12/1
  [dout] -> first/1, second/1
  d/1 -> reorder/3(din0)  "di"
  [valid] -> Logical3/1, Logical1/2, Logical/2, addr/2  "v1"
  Delay5/1 -> Terminator/1
  Delay4/1 -> Delay5/1
  Delay2/1 -> Mux2/3
  Delay1/1 -> Mux2/2
  Mux2/1 -> [add]  "add"
  [lsb] -> Logical/1, Inverter1/1, Logical3/2
  Slice1/1 -> [lsb]
  Slice3/1 -> Delay2/1, col_sel/1, row_sel/1, buffer/1
  Inverter1/1 -> Logical1/1
  Logical3/1 -> [pre], Delay3/1
  Delay6/1 -> [win]  "win"
  first/1 -> Mux1/3  "first"
  second/1 -> Mux1/2  "second"
  col_sel/1 -> Concat/3
  edge_detect1/1(out) -> Register4/3, Register4/1
  [buffer] -> edge_detect1/1(in)
  Delay3/1 -> Delay6/1, [rin]  "rin"
  Inverter2/1 -> Concat/1
  Concat/1 -> Delay1/1
  [rin] -> Mux2/1
  row_sel/1 -> Concat/2
  edge_detect/1(out) -> sync_delay/1
  Register2/1 -> edge_detect/1(in)
  Logical6/1 -> Register4/2, Register2/2
  [pre] -> Logical6/2
  Register4/1 -> Logical6/1
  [sync] -> Register2/3, Register2/1
  buffer/1 -> Delay4/1, Inverter2/1, [buffer]
  [din] -> qdr/5  "din"
  Mux1/1 -> [din]  "din"
  [rin] -> Mux1/1
  Logical1/1 -> first/2
  Logical/1 -> second/2
  addr/1 -> Slice3/1, Slice1/1
  qdr/3 -> Terminator2/1
  qdr/4 -> Inverter7/1
  qdr/5 -> Logical12/2
  [add] -> qdr/4, Register1/1, Relational/1  "addr"
  Constant/1 -> qdr/3
  [win] -> qdr/2  "win"
  [rin] -> qdr/1  "rin"
  en/1 -> reorder/2(en)  "vi"
  sync/1 -> reorder/1(sync)  "si"
